simulink model "ECmodel2"  (R2014a)
settings: Solver=ode45  StartTime=0.0  StopTime=4200  RelTol=1e-3
settings Model: Creator=Suda  LastModifiedBy=Suda

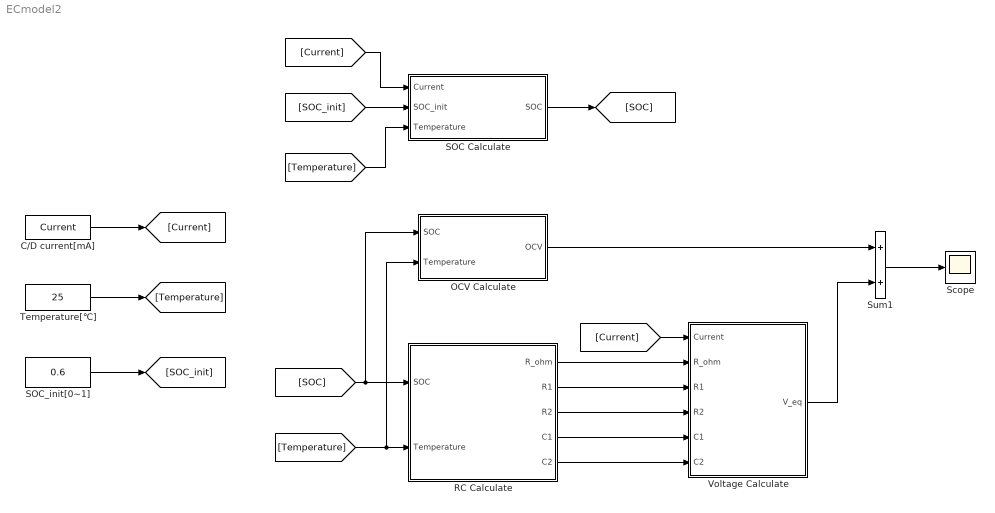
== system ECmodel2 ==
  C/D current[mA] : FromWorkspace  VariableName=Current  SampleTime=0
  OCV Calculate : Subsystem
  RC Calculate : Subsystem
  SOC Calculate : Subsystem
  SOC_init[0~1] : Constant  Value=0.6
  Scope : Scope
  Sum1 : Sum
  Temperature[℃] : Constant  Value=25
  Voltage Calculate : Subsystem
  wires:
  OCV Calculate/1(OCV) -> Sum1/1
  RC Calculate/1(R_ohm) -> Voltage Calculate/2("R_ohm ")
  RC Calculate/2(R1) -> Voltage Calculate/3(R1)
  RC Calculate/3(R2) -> Voltage Calculate/4(R2)
  RC Calculate/4(C1) -> Voltage Calculate/5(C1)
  RC Calculate/5(C2) -> Voltage Calculate/6(C2)
  Voltage Calculate/1(V_eq) -> Sum1/2
  Sum1/1 -> Scope/1
  C/D current[mA]/1 -> [Current]
  [Current] -> SOC Calculate/1(Current)
  Temperature[℃]/1 -> [Temperature]
  [Temperature] -> SOC Calculate/3("Temperature ")
  SOC Calculate/1(SOC) -> [SOC]
  [Temperature] -> OCV Calculate/2(Temperature), RC Calculate/2(Temperature)
  [Current] -> Voltage Calculate/1(Current)
  [SOC] -> RC Calculate/1(SOC), OCV Calculate/1(SOC)
  SOC_init[0~1]/1 -> [SOC_init]
  [SOC_init] -> SOC Calculate/2(SOC_init)

== system ECmodel2/OCV Calculate ==
  SOC : Inport
  Temperature : Inport  Port=2
  -10℃ : Subsystem
  10℃ : Subsystem
  25℃ : Subsystem
  40℃ : Subsystem
  55℃ : Subsystem
  Chart : Stateflow chart  TreatAsAtomicUnit=on
  OCV : Outport
  wires:
  SOC/1 -> 55℃/1(SOC), 40℃/1(SOC), 25℃/1(SOC), 10℃/1(SOC), -10℃/1(SOC)
  Temperature/1 -> Chart/1(T)
  -10℃/1(OCV_-10) -> Chart/2(OCV_N10)
  10℃/1(OCV_10) -> Chart/3(OCV_10)
  25℃/1(OCV_25) -> Chart/4(OCV_25)
  40℃/1(OCV_40) -> Chart/5(OCV_40)
  55℃/1(OCV_55) -> Chart/6(OCV_55)
  Chart/1(OCV) -> OCV/1

== system ECmodel2/RC Calculate ==
  SOC : Inport
  Temperature : Inport  Port=2
  Subsystem : Subsystem
  Subsystem1 : Subsystem
  Subsystem2 : Subsystem
  Subsystem3 : Subsystem
  Subsystem4 : Subsystem
  R_ohm : Outport
  R1 : Outport  Port=2
  R2 : Outport  Port=3
  C1 : Outport  Port=4
  C2 : Outport  Port=5
  wires:
  Temperature/1 -> Subsystem4/1(Tempearture), Subsystem3/1(Temperature), Subsystem2/1(Temperature), Subsystem1/1(Tempearture), Subsystem/2(Temperature)
  Subsystem/1(R_ohm) -> R_ohm/1
  Subsystem1/1(R1) -> R1/1
  Subsystem2/1(C1) -> C1/1
  Subsystem3/1(R2) -> R2/1
  Subsystem4/1(C2) -> C2/1
  SOC/1 -> Subsystem/1(SOC)

== system ECmodel2/SOC Calculate ==
  Current : Inport
  SOC_init : Inport  Port=2
  "Temperature " : Inport  Port=3
  "  " : Product  Inputs=*/
  "    " : Product
  Capacity Calculate : Subsystem
  Constant : Constant  Value=3600
  Integrator : Integrator
  Sum : Sum  Inputs=|++
  SOC : Outport
  wires:
  "Temperature "/1 -> Capacity Calculate/1(Temperature)
  "    "/1 -> "  "/2
  Integrator/1 -> Sum/1
  SOC_init/1 -> Sum/2
  "  "/1 -> Integrator/1
  Current/1 -> "  "/1
  Capacity Calculate/1(Capacity[mAh]) -> "    "/1
  Constant/1 -> "    "/2
  Sum/1 -> SOC/1

== system ECmodel2/Voltage Calculate ==
  Current : Inport
  "R_ohm " : Inport  Port=2
  R1 : Inport  Port=3
  R2 : Inport  Port=4
  C1 : Inport  Port=5
  C2 : Inport  Port=6
  Product : Product
  Subsystem : Subsystem
  Subsystem1 : Subsystem
  Sum : Sum  Inputs=+++
  V_eq : Outport
  wires:
  "R_ohm "/1 -> Product/1
  Product/1 -> Sum/1
  Sum/1 -> V_eq/1
  Current/1 -> Subsystem1/2(Current), Subsystem/2(Current), Product/2
  C1/1 -> Subsystem/1(C1)
  R1/1 -> Subsystem/3(R1)
  Subsystem/1(V1) -> Sum/2
  C2/1 -> Subsystem1/1(C2)
  R2/1 -> Subsystem1/3(R2)
  Subsystem1/1(V2) -> Sum/3

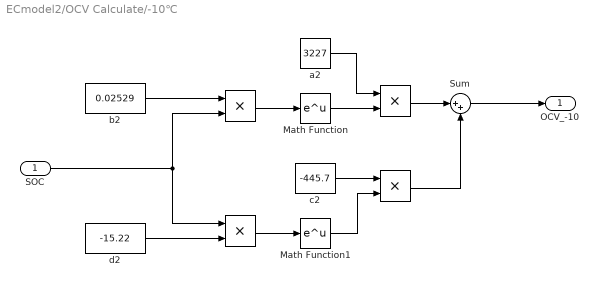
== system ECmodel2/OCV Calculate/-10℃ ==
  SOC : Inport
  " " : Product
  "  " : Product
  "   " : Product
  "    " : Product
  Math Function : Math  SaturateOnIntegerOverflow=on
  Math Function1 : Math  SaturateOnIntegerOverflow=on
  Sum : Sum  Inputs=|++
  a2 : Constant  Value=3227
  b2 : Constant  Value=0.02529
  c2 : Constant  Value=-445.7
  d2 : Constant  Value=-15.22
  OCV_-10 : Outport
  wires:
  Sum/1 -> OCV_-10/1
  d2/1 -> "  "/2
  SOC/1 -> " "/2, "  "/1
  " "/1 -> Math Function/1
  Math Function1/1 -> "    "/2
  "  "/1 -> Math Function1/1
  Math Function/1 -> "   "/2
  c2/1 -> "    "/1
  "   "/1 -> Sum/1
  "    "/1 -> Sum/2
  b2/1 -> " "/1
  a2/1 -> "   "/1

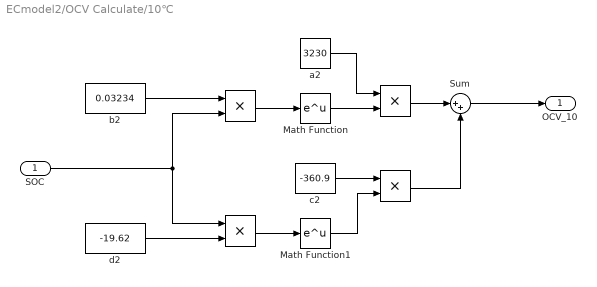
== system ECmodel2/OCV Calculate/10℃ ==
  SOC : Inport
  " " : Product
  "  " : Product
  "   " : Product
  "    " : Product
  Math Function : Math  SaturateOnIntegerOverflow=on
  Math Function1 : Math  SaturateOnIntegerOverflow=on
  Sum : Sum  Inputs=|++
  a2 : Constant  Value=3230
  b2 : Constant  Value=0.03234
  c2 : Constant  Value=-360.9
  d2 : Constant  Value=-19.62
  OCV_10 : Outport
  wires:
  Sum/1 -> OCV_10/1
  d2/1 -> "  "/2
  SOC/1 -> " "/2, "  "/1
  " "/1 -> Math Function/1
  Math Function1/1 -> "    "/2
  "  "/1 -> Math Function1/1
  Math Function/1 -> "   "/2
  c2/1 -> "    "/1
  "   "/1 -> Sum/1
  "    "/1 -> Sum/2
  b2/1 -> " "/1
  a2/1 -> "   "/1

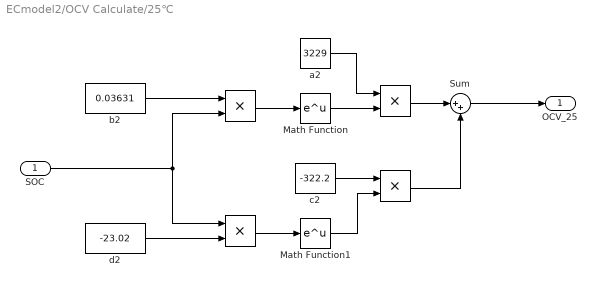
== system ECmodel2/OCV Calculate/25℃ ==
  SOC : Inport
  " " : Product
  "  " : Product
  "   " : Product
  "    " : Product
  Math Function : Math  SaturateOnIntegerOverflow=on
  Math Function1 : Math  SaturateOnIntegerOverflow=on
  Sum : Sum  Inputs=|++
  a2 : Constant  Value=3229
  b2 : Constant  Value=0.03631
  c2 : Constant  Value=-322.2
  d2 : Constant  Value=-23.02
  OCV_25 : Outport
  wires:
  Sum/1 -> OCV_25/1
  d2/1 -> "  "/2
  SOC/1 -> " "/2, "  "/1
  " "/1 -> Math Function/1
  Math Function1/1 -> "    "/2
  "  "/1 -> Math Function1/1
  Math Function/1 -> "   "/2
  c2/1 -> "    "/1
  "   "/1 -> Sum/1
  "    "/1 -> Sum/2
  b2/1 -> " "/1
  a2/1 -> "   "/1

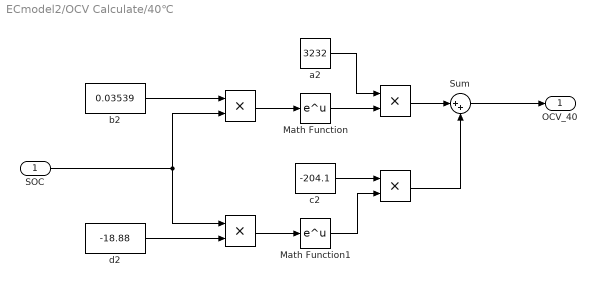
== system ECmodel2/OCV Calculate/40℃ ==
  SOC : Inport
  " " : Product
  "  " : Product
  "   " : Product
  "    " : Product
  Math Function : Math  SaturateOnIntegerOverflow=on
  Math Function1 : Math  SaturateOnIntegerOverflow=on
  Sum : Sum  Inputs=|++
  a2 : Constant  Value=3232
  b2 : Constant  Value=0.03539
  c2 : Constant  Value=-204.1
  d2 : Constant  Value=-18.88
  OCV_40 : Outport
  wires:
  Sum/1 -> OCV_40/1
  d2/1 -> "  "/2
  SOC/1 -> " "/2, "  "/1
  " "/1 -> Math Function/1
  Math Function1/1 -> "    "/2
  "  "/1 -> Math Function1/1
  Math Function/1 -> "   "/2
  c2/1 -> "    "/1
  "   "/1 -> Sum/1
  "    "/1 -> Sum/2
  b2/1 -> " "/1
  a2/1 -> "   "/1

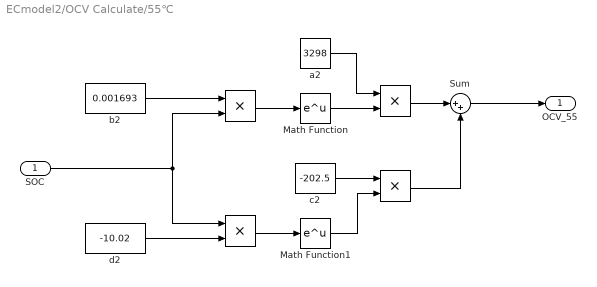
== system ECmodel2/OCV Calculate/55℃ ==
  SOC : Inport
  " " : Product
  "  " : Product
  "   " : Product
  "    " : Product
  Math Function : Math  SaturateOnIntegerOverflow=on
  Math Function1 : Math  SaturateOnIntegerOverflow=on
  Sum : Sum  Inputs=|++
  a2 : Constant  Value=3298
  b2 : Constant  Value=0.001693
  c2 : Constant  Value=-202.5
  d2 : Constant  Value=-10.02
  OCV_55 : Outport
  wires:
  Sum/1 -> OCV_55/1
  d2/1 -> "  "/2
  SOC/1 -> " "/2, "  "/1
  " "/1 -> Math Function/1
  Math Function1/1 -> "    "/2
  "  "/1 -> Math Function1/1
  Math Function/1 -> "   "/2
  c2/1 -> "    "/1
  "   "/1 -> Sum/1
  "    "/1 -> Sum/2
  b2/1 -> " "/1
  a2/1 -> "   "/1

== system ECmodel2/RC Calculate/Subsystem ==
  SOC : Inport
  Temperature : Inport  Port=2
  -10℃ : Subsystem
  10℃ : Subsystem
  25℃ : Subsystem
  40℃ : Subsystem
  55℃ : Subsystem
  Chart : Stateflow chart  TreatAsAtomicUnit=on
  R_ohm : Outport
  wires:
  Temperature/1 -> Chart/1(T)
  -10℃/1(ohm_-10) -> Chart/2(ohm_N10)
  10℃/1(ohm_10) -> Chart/3(ohm_10)
  25℃/1(ohm_25) -> Chart/4(ohm_25)
  40℃/1(ohm_40) -> Chart/5(ohm_40)
  55℃/1(ohm_55) -> Chart/6(ohm_55)
  Chart/1(R_ohm) -> R_ohm/1
  SOC/1 -> 55℃/1(SOC), 40℃/1(SOC), 25℃/1(SOC), 10℃/1(SOC), -10℃/1(SOC)

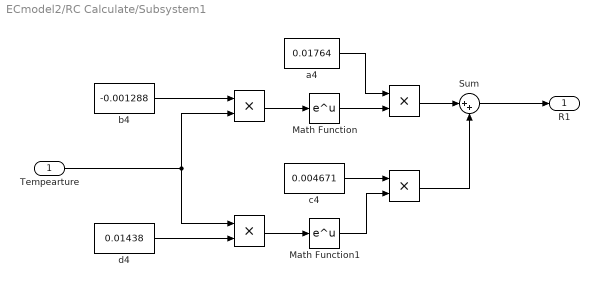
== system ECmodel2/RC Calculate/Subsystem1 ==
  Tempearture : Inport
  " " : Product
  "  " : Product
  "   " : Product
  "    " : Product
  Math Function : Math  SaturateOnIntegerOverflow=on
  Math Function1 : Math  SaturateOnIntegerOverflow=on
  Sum : Sum  Inputs=|++
  a4 : Constant  Value=0.01764
  b4 : Constant  Value=-0.001288
  c4 : Constant  Value=0.004671
  d4 : Constant  Value=0.01438
  R1 : Outport
  wires:
  Sum/1 -> R1/1
  d4/1 -> "  "/2
  Tempearture/1 -> " "/2, "  "/1
  " "/1 -> Math Function/1
  Math Function1/1 -> "    "/2
  "  "/1 -> Math Function1/1
  Math Function/1 -> "   "/2
  c4/1 -> "    "/1
  "   "/1 -> Sum/1
  "    "/1 -> Sum/2
  b4/1 -> " "/1
  a4/1 -> "   "/1

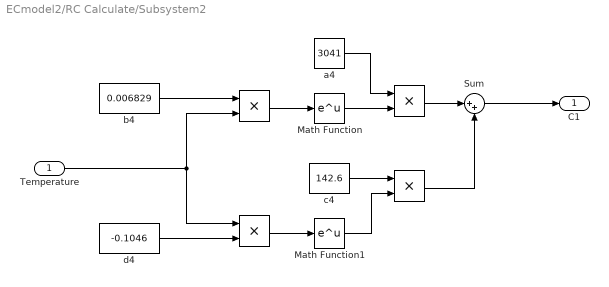
== system ECmodel2/RC Calculate/Subsystem2 ==
  Temperature : Inport
  " " : Product
  "  " : Product
  "   " : Product
  "    " : Product
  Math Function : Math  SaturateOnIntegerOverflow=on
  Math Function1 : Math  SaturateOnIntegerOverflow=on
  Sum : Sum  Inputs=|++
  a4 : Constant  Value=3041
  b4 : Constant  Value=0.006829
  c4 : Constant  Value=142.6
  d4 : Constant  Value=-0.1046
  C1 : Outport
  wires:
  Sum/1 -> C1/1
  d4/1 -> "  "/2
  Temperature/1 -> " "/2, "  "/1
  " "/1 -> Math Function/1
  Math Function1/1 -> "    "/2
  "  "/1 -> Math Function1/1
  Math Function/1 -> "   "/2
  c4/1 -> "    "/1
  "   "/1 -> Sum/1
  "    "/1 -> Sum/2
  b4/1 -> " "/1
  a4/1 -> "   "/1

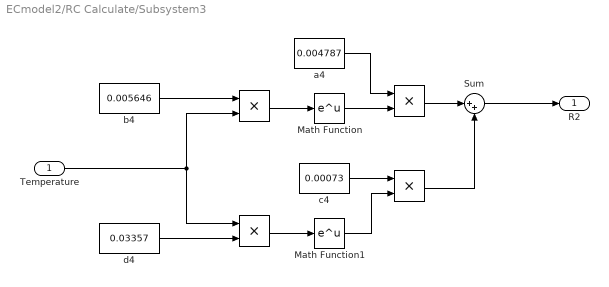
== system ECmodel2/RC Calculate/Subsystem3 ==
  Temperature : Inport
  " " : Product
  "  " : Product
  "   " : Product
  "    " : Product
  Math Function : Math  SaturateOnIntegerOverflow=on
  Math Function1 : Math  SaturateOnIntegerOverflow=on
  Sum : Sum  Inputs=|++
  a4 : Constant  Value=0.004787
  b4 : Constant  Value=0.005646
  c4 : Constant  Value=0.00073
  d4 : Constant  Value=0.03357
  R2 : Outport
  wires:
  Sum/1 -> R2/1
  d4/1 -> "  "/2
  Temperature/1 -> " "/2, "  "/1
  " "/1 -> Math Function/1
  Math Function1/1 -> "    "/2
  "  "/1 -> Math Function1/1
  Math Function/1 -> "   "/2
  c4/1 -> "    "/1
  "   "/1 -> Sum/1
  "    "/1 -> Sum/2
  b4/1 -> " "/1
  a4/1 -> "   "/1

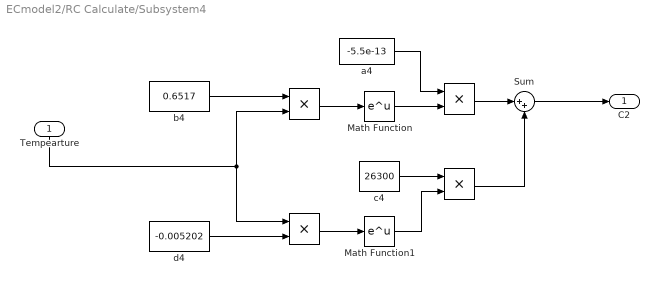
== system ECmodel2/RC Calculate/Subsystem4 ==
  Tempearture : Inport
  " " : Product
  "  " : Product
  "   " : Product
  "    " : Product
  Math Function : Math  SaturateOnIntegerOverflow=on
  Math Function1 : Math  SaturateOnIntegerOverflow=on
  Sum : Sum  Inputs=|++
  a4 : Constant  Value=-5.5e-13
  b4 : Constant  Value=0.6517
  c4 : Constant  Value=26300
  d4 : Constant  Value=-0.005202
  C2 : Outport
  wires:
  Sum/1 -> C2/1
  d4/1 -> "  "/2
  Tempearture/1 -> " "/2, "  "/1
  " "/1 -> Math Function/1
  Math Function1/1 -> "    "/2
  "  "/1 -> Math Function1/1
  Math Function/1 -> "   "/2
  c4/1 -> "    "/1
  "   "/1 -> Sum/1
  "    "/1 -> Sum/2
  b4/1 -> " "/1
  a4/1 -> "   "/1

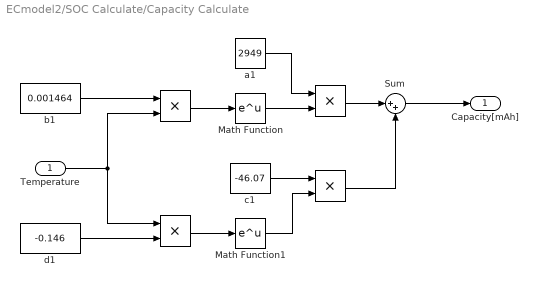
== system ECmodel2/SOC Calculate/Capacity Calculate ==
  Temperature : Inport
  " " : Product
  "  " : Product
  "   " : Product
  "    " : Product
  Math Function : Math  SaturateOnIntegerOverflow=on
  Math Function1 : Math  SaturateOnIntegerOverflow=on
  Sum : Sum  Inputs=|++
  a1 : Constant  Value=2949
  b1 : Constant  Value=0.001464
  c1 : Constant  Value=-46.07
  d1 : Constant  Value=-0.146
  Capacity[mAh] : Outport
  wires:
  d1/1 -> "  "/2
  Sum/1 -> Capacity[mAh]/1
  Temperature/1 -> " "/2, "  "/1
  "    "/1 -> Sum/2
  b1/1 -> " "/1
  Math Function/1 -> "   "/2
  " "/1 -> Math Function/1
  Math Function1/1 -> "    "/2
  "  "/1 -> Math Function1/1
  c1/1 -> "    "/1
  "   "/1 -> Sum/1
  a1/1 -> "   "/1

== system ECmodel2/Voltage Calculate/Subsystem ==
  C1 : Inport
  Current : Inport  Port=2
  R1 : Inport  Port=3
  Fcn : Fcn  Expr=1/u
  Fcn1 : Fcn  Expr=1/u
  Integrator : Integrator
  Product2 : Product
  Product3 : Product
  Sum1 : Sum  Inputs=|+-
  V1 : Outport
  wires:
  Current/1 -> Sum1/1
  Fcn1/1 -> Product3/2
  Product3/1 -> Sum1/2
  Fcn/1 -> Product2/1
  Sum1/1 -> Product2/2
  C1/1 -> Fcn/1
  Product2/1 -> Integrator/1
  R1/1 -> Fcn1/1
  Integrator/1 -> V1/1, Product3/1

== system ECmodel2/Voltage Calculate/Subsystem1 ==
  C2 : Inport
  Current : Inport  Port=2
  R2 : Inport  Port=3
  Fcn2 : Fcn  Expr=1/u
  Fcn3 : Fcn  Expr=1/u
  Integrator1 : Integrator
  Product4 : Product
  Product5 : Product
  Sum2 : Sum  Inputs=|+-
  V2 : Outport
  wires:
  Current/1 -> Sum2/1
  Sum2/1 -> Product4/2
  C2/1 -> Fcn2/1
  Fcn2/1 -> Product4/1
  R2/1 -> Fcn3/1
  Product4/1 -> Integrator1/1
  Integrator1/1 -> V2/1, Product5/1
  Fcn3/1 -> Product5/2
  Product5/1 -> Sum2/2

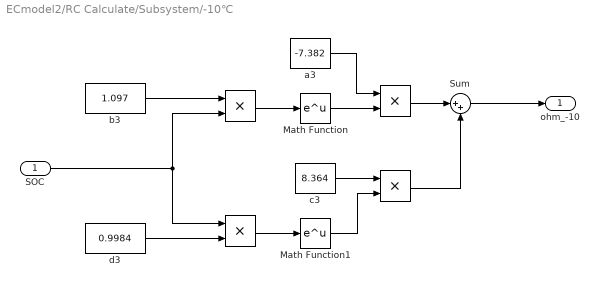
== system ECmodel2/RC Calculate/Subsystem/-10℃ ==
  SOC : Inport
  " " : Product
  "  " : Product
  "   " : Product
  "    " : Product
  Math Function : Math  SaturateOnIntegerOverflow=on
  Math Function1 : Math  SaturateOnIntegerOverflow=on
  Sum : Sum  Inputs=|++
  a3 : Constant  Value=-7.382
  b3 : Constant  Value=1.097
  c3 : Constant  Value=8.364
  d3 : Constant  Value=0.9984
  ohm_-10 : Outport
  wires:
  Sum/1 -> ohm_-10/1
  d3/1 -> "  "/2
  SOC/1 -> " "/2, "  "/1
  " "/1 -> Math Function/1
  Math Function1/1 -> "    "/2
  "  "/1 -> Math Function1/1
  Math Function/1 -> "   "/2
  c3/1 -> "    "/1
  "   "/1 -> Sum/1
  "    "/1 -> Sum/2
  b3/1 -> " "/1
  a3/1 -> "   "/1

== system ECmodel2/RC Calculate/Subsystem/10℃ ==
  SOC : Inport
  " " : Product
  "  " : Product
  "   " : Product
  "    " : Product
  Math Function : Math  SaturateOnIntegerOverflow=on
  Math Function1 : Math  SaturateOnIntegerOverflow=on
  Sum : Sum  Inputs=|++
  a3 : Constant  Value=0.1901
  b3 : Constant  Value=-0.4899
  c3 : Constant  Value=0.09331
  d3 : Constant  Value=0.434
  ohm_10 : Outport
  wires:
  Sum/1 -> ohm_10/1
  d3/1 -> "  "/2
  SOC/1 -> " "/2, "  "/1
  " "/1 -> Math Function/1
  Math Function1/1 -> "    "/2
  "  "/1 -> Math Function1/1
  Math Function/1 -> "   "/2
  c3/1 -> "    "/1
  "   "/1 -> Sum/1
  "    "/1 -> Sum/2
  b3/1 -> " "/1
  a3/1 -> "   "/1

== system ECmodel2/RC Calculate/Subsystem/25℃ ==
  SOC : Inport
  " " : Product
  "  " : Product
  "   " : Product
  "    " : Product
  Math Function : Math  SaturateOnIntegerOverflow=on
  Math Function1 : Math  SaturateOnIntegerOverflow=on
  Sum : Sum  Inputs=|++
  a3 : Constant  Value=0.0151
  b3 : Constant  Value=-2.504
  c3 : Constant  Value=0.2302
  d3 : Constant  Value=-0.00124
  ohm_25 : Outport
  wires:
  Sum/1 -> ohm_25/1
  d3/1 -> "  "/2
  SOC/1 -> " "/2, "  "/1
  " "/1 -> Math Function/1
  Math Function1/1 -> "    "/2
  "  "/1 -> Math Function1/1
  Math Function/1 -> "   "/2
  c3/1 -> "    "/1
  "   "/1 -> Sum/1
  "    "/1 -> Sum/2
  b3/1 -> " "/1
  a3/1 -> "   "/1

== system ECmodel2/RC Calculate/Subsystem/40℃ ==
  SOC : Inport
  " " : Product
  "  " : Product
  "   " : Product
  "    " : Product
  Math Function : Math  SaturateOnIntegerOverflow=on
  Math Function1 : Math  SaturateOnIntegerOverflow=on
  Sum : Sum  Inputs=|++
  a3 : Constant  Value=0.008852
  b3 : Constant  Value=-10.72
  c3 : Constant  Value=0.2487
  d3 : Constant  Value=-0.02033
  ohm_40 : Outport
  wires:
  Sum/1 -> ohm_40/1
  d3/1 -> "  "/2
  SOC/1 -> " "/2, "  "/1
  " "/1 -> Math Function/1
  Math Function1/1 -> "    "/2
  "  "/1 -> Math Function1/1
  Math Function/1 -> "   "/2
  c3/1 -> "    "/1
  "   "/1 -> Sum/1
  "    "/1 -> Sum/2
  b3/1 -> " "/1
  a3/1 -> "   "/1

== system ECmodel2/RC Calculate/Subsystem/55℃ ==
  SOC : Inport
  " " : Product
  "  " : Product
  "   " : Product
  "    " : Product
  Math Function : Math  SaturateOnIntegerOverflow=on
  Math Function1 : Math  SaturateOnIntegerOverflow=on
  Sum : Sum  Inputs=|++
  a3 : Constant  Value=0.003233
  b3 : Constant  Value=-3.733
  c3 : Constant  Value=0.297
  d3 : Constant  Value=-0.03979
  ohm_55 : Outport
  wires:
  Sum/1 -> ohm_55/1
  d3/1 -> "  "/2
  SOC/1 -> " "/2, "  "/1
  " "/1 -> Math Function/1
  Math Function1/1 -> "    "/2
  "  "/1 -> Math Function1/1
  Math Function/1 -> "   "/2
  c3/1 -> "    "/1
  "   "/1 -> Sum/1
  "    "/1 -> Sum/2
  b3/1 -> " "/1
  a3/1 -> "   "/1

== stateflow chart ECmodel2/RC Calculate/Subsystem/Chart ==
  (default) -> (junction 14)
  (junction 14) -> (junction 15) [order 1] : [T>10]
  (junction 15) -> (junction 16) [order 1] : [T>25]
  (junction 16) -> (junction 29) [order 1] : [T>40]
  (junction 29) -> (junction 34) [order 1] : [T>55]
  (junction 14) -> (junction 10) [order 2] : {R_ohm=ohm_N10+(ohm_10-ohm_N10)*(T+10)/20}
  (junction 15) -> (junction 18) [order 2] : {R_ohm=ohm_10+(ohm_25-ohm_10)*(T-10)/15}
  (junction 16) -> (junction 19) [order 2] : {R_ohm=ohm_25+(ohm_40-ohm_25)*(T-25)/15}
  (junction 29) -> (junction 30) [order 2] : {R_ohm=ohm_40+(ohm_55-ohm_40)*(T-40)/15}
  (junction 34) -> (junction 36) : {R_ohm=ohm_55+(ohm_55-ohm_40)*(T-55)/15}
  (junction 18) -> (junction 10)
  (junction 19) -> (junction 18)
  (junction 30) -> (junction 19)
  (junction 36) -> (junction 30)
  (junction 10) -> (junction 11)
  data: T input [-20..60]; ohm_N10 input; ohm_10 input; ohm_25 input; ohm_40 input; ohm_55 input; R_ohm output

== stateflow chart ECmodel2/OCV Calculate/Chart ==
  (default) -> (junction 14)
  (junction 14) -> (junction 15) [order 1] : [T>10]
  (junction 15) -> (junction 16) [order 1] : [T>25]
  (junction 16) -> (junction 29) [order 1] : [T>40]
  (junction 29) -> (junction 34) [order 1] : [T>55]
  (junction 14) -> (junction 10) [order 2] : {OCV=OCV_N10+(OCV_10-OCV_N10)*(T+10)/20}
  (junction 15) -> (junction 18) [order 2] : {OCV=OCV_10+(OCV_25-OCV_10)*(T-10)/15}
  (junction 16) -> (junction 19) [order 2] : {OCV=OCV_25+(OCV_40-OCV_25)*(T-25)/15}
  (junction 29) -> (junction 30) [order 2] : {OCV=OCV_40+(OCV_55-OCV_40)*(T-40)/15}
  (junction 34) -> (junction 36) : {OCV=OCV_55+(OCV_55-OCV_40)*(T-55)/15}
  (junction 18) -> (junction 10)
  (junction 19) -> (junction 18)
  (junction 30) -> (junction 19)
  (junction 36) -> (junction 30)
  (junction 10) -> (junction 11)
  data: T input [-20..60]; OCV_N10 input; OCV_10 input; OCV_25 input; OCV_40 input; OCV_55 input; OCV output
